simulink model "Engine_TestBench1"  (R2017a)
settings: Solver=ode1  StartTime=0.0  StopTime=1800  FixedStep=0.01  RelTol=1e-3  EnableMultiTasking=on
PostLoadFcn:
  | , if any(exist('dsrtsu_mdlpostloadfcn', 'file') == [2, 3, 6]), try dsrtsu_mdlpostloadfcn('Execute', bdroot); catch fprintf('Error in PostLoadFcn (dsrtsu_mdlpostloadfcn) for model "%s":\n %s\n', bdroot, lasterr); end, end,
undefined symbols (not defined in the file): air, Engine, env, max_vehicle_rad_air_flow, NeutralGear, ParkGear
libraries: simulink x19, EC2_libraries x2
(part 1 of 2)
settings Model: DSRTSU_INTERNAL_RTI_VER=480  DSRTSU_INTERNAL_RTI_TYPE=rti1006  RTICANMMDATA=struct('GeneralSetupData',struct('modelroot','D:\Desktop_files\Clutchless_P2_Model_R2015b','generalsettings',struct('filesettings',struct('destfolder',struct('Name','RTICANMM_FILES','Check',1),'buildfolder',struct('Name','.','Check',1),'AbsDestfolder',struct('Name','D:\Desktop_files\Clutchless_P2_Model_R2015b\RTICANMM_FILES'),'AbsBuildfolder',struct('Name','D:\Desktop_files\Clutchless_P2_Model_R2015b'))),'options',struct('addpaths',1,'rmpaths',1,'addtrcexclusion',logical(1),'cannavigator',struct('checkmonitoring',0),'show_usrtrc',0,'use_usrtrc',0),'advanced',struct('options',[1 1 1 1 1 1 1 1 1 1 1 1 1 1 1 1 1 1 1 1 1 1 1 1 1 1 1 1 1 1 1 1 1 1 1 1 1 1 1 1 1 1 1 1 1 1 1 1 1 1 1 1 1 1 1 1 1 1 1 1 1 1 1 1 1 1 1 1 1 1 1 1 1 1 1 1 1 1 1 1 1 1 1 1 1 1 1 1 1 1 1 1 1 1 1 1 1 1 1 1]),'MPSetup',{{}},'modelname','P2_Parallel_MIL_withTrailer','block','P2_Parallel_MIL_withTrailer'))  DSRTSU_INTERNAL_RTIFPGA=70  SimulationMode=accelerator  Creator=EcoCar  LastModifiedBy=Vraj M
settings DataIOCC: LimitDataPoints=on
settings OptimizationCC: BlockReduction=off  OptimizeBlockIOStorage=off  BufferReuse=off  GlobalBufferReuse=off  ExpressionFolding=off  LocalBlockOutputs=off  EfficientMapNaN2IntZero=off  LifeSpan=inf
settings DebuggingCC: AllowSymbolicDim=off  SFUnexpectedBacktrackingDiag=warning  SFNoUnconditionalDefaultTransitionDiag=warning  SFExecutionAtInitializationDiag=none
settings HardwareCC: ProdBitPerPointer=32  ProdBitPerSizeT=32  ProdBitPerPtrDiffT=32  ProdLargestAtomicInteger=Integer  ProdWordSize=32  ProdHWDeviceType=Custom Processor->Custom  TargetBitPerPointer=64  TargetBitPerSizeT=64  TargetBitPerPtrDiffT=64  TargetLongLongMode=on  TargetIntDivRoundTo=Zero  TargetEndianess=LittleEndian  TargetWordSize=64  TargetHWDeviceType=MATLAB Host  ProdEqTarget=off
settings ModelReferenceCC: PropagateSignalLabelsOutOfModel=off
settings CodeAppCC: MaxIdLength=128
settings GRTTargetCC: TargetLangStandard=C89/C90 (ANSI)  CombineOutputUpdateFcns=off  GRTInterface=on
settings ConfigComp: CovScope=ReferencedModels  CovIncludeTopModel=off  CovMetricSettings=dw  CovHtmlReporting=on  CovSaveCumulativeToWorkspaceVar=on  CovSaveSingleToWorkspaceVar=on  CovExternalEMLEnable=off

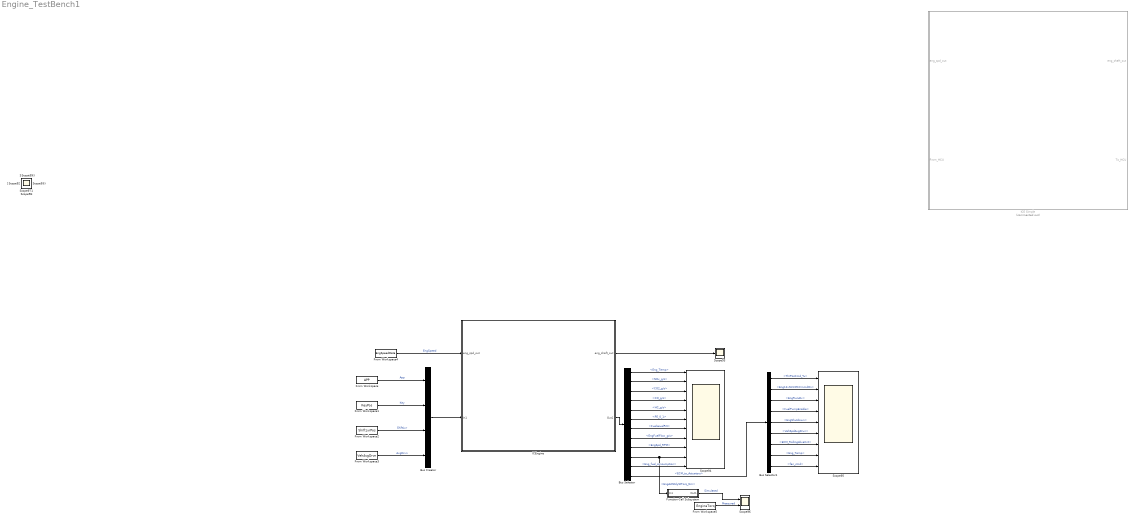
== system Engine_TestBench1 ==
  Bus Creator : BusCreator  Inputs=4
  Bus Selector : BusSelector  OutputSignals=Sensors_to_ECM.Eng_Temp,Sensors_to_ECM.NOx_g/s,Sensors_to_ECM.CO2_g/s,Sensors_to_ECM.CO_g/s,Sensors_to_ECM.HC_g/s,Sensors_to_ECM.PE_0_1,Sensors_to_ECM.FuelLevelPct,Sensors_to_ECM.EngFuelFlow_g/s,Sensors_to_ECM.EngSpd_RPM,Sensors_to_ECM.EngActStdyStTorq_Nm,Eng_fuel_consumption,ECM_to_Actuators
  Bus Selector1 : BusSelector  OutputSignals=ThrPosCmd_%,Eng12vStrtrMtrCmmdOn,EngRunAtv,FuelPumpEnable,EngShutdown,VehSpdAvgDrvn,ECM_RollingAliveCnt,Eng_Temp,fan_cmd
  From Workspace : FromWorkspace  VariableName=APP  SampleTime=0
  From Workspace1 : FromWorkspace  VariableName=KeyPos  SampleTime=0
  From Workspace2 : FromWorkspace  VariableName=ShiftLvrPos  SampleTime=0
  From Workspace3 : FromWorkspace  VariableName=VehAvgDrvn  SampleTime=0
  From Workspace4 : FromWorkspace  VariableName=EngSpeedData  SampleTime=0
  From Workspace5 : FromWorkspace  VariableName=EngineTorq  SampleTime=0
  Function-Call Subsystem : Subsystem  TreatAsAtomicUnit=on
  ICE Simple : Subsystem  Commented=on  AncestorBlock=Engine_simple/ICE Simple
      mask Display:
      | image(imread('EngineTopLevel.jpg'),'center')
      | color('red');
      | port_label('input',1,'SpdOut')
      | port_label('output',1,'ShaftOut')
      | port_label('input',2,'From_HCU')
      | port_label('output',2,'To_HCU')
  ICEngine : Subsystem  AncestorBlock=Engine_simple/ICE Simple
      mask Display:
      | image(imread('EngineTopLevel.jpg'),'center')
      | color('red');
      | port_label('input',1,'SpdOut')
      | port_label('output',1,'ShaftOut')
  Scope{,1..93,97..105} (103 alike) : Scope
  Scope94 : Scope  NumInputPorts=11
  Scope95 : Scope  NumInputPorts=9
  Scope96 : Scope  NumInputPorts=2
  wires:
  Bus Selector1/4 -> Scope95/4  "<FuelPumpEnable>"
  From Workspace2/1 -> Bus Creator/3  "ShiftLvr"
  From Workspace4/1 -> ICEngine/1(eng_spd_out)  "EngSpeed"
  Bus Selector1/7 -> Scope95/7  "<ECM_RollingAliveCnt>"
  ICEngine/2(Out1) -> Bus Selector/1
  Bus Selector1/8 -> Scope95/8  "<Eng_Temp>"
  From Workspace1/1 -> Bus Creator/2  "Key"
  Bus Selector/7 -> Scope94/7  "<FuelLevelPct>"
  Bus Selector/4 -> Scope94/4  "<CO_g/s>"
  Bus Selector/9 -> Scope94/9  "<EngSpd_RPM>"
  Bus Selector/5 -> Scope94/5  "<HC_g/s>"
  Bus Selector/6 -> Scope94/6  "<PE_0_1>"
  Bus Selector/3 -> Scope94/3  "<CO2_g/s>"
  Bus Selector/2 -> Scope94/2  "<NOx_g/s>"
  Bus Selector/10 -> Function-Call Subsystem/1(In1), Scope94/10  "<EngActStdyStTorq_Nm>"
  Bus Selector/11 -> Scope94/11  "<Eng_fuel_consumption>"
  Bus Selector1/6 -> Scope95/6  "<VehSpdAvgDrvn>"
  Bus Creator/1 -> ICEngine/2(In1)
  Bus Selector1/2 -> Scope95/2  "<Eng12vStrtrMtrCmmdOn>"
  Bus Selector1/9 -> Scope95/9  "<fan_cmd>"
  Bus Selector1/1 -> Scope95/1  "<ThrPosCmd_%>"
  Bus Selector1/3 -> Scope95/3  "<EngRunAtv>"
  Bus Selector/1 -> Scope94/1  "<Eng_Temp>"
  From Workspace3/1 -> Bus Creator/4  "AvgDrvn"
  Bus Selector/12 -> Bus Selector1/1  "<ECM_to_Actuators>"
  ICEngine/1(eng_shaft_out) -> Scope93/1
  Bus Selector1/5 -> Scope95/5  "<EngShutdown>"
  Bus Selector/8 -> Scope94/8  "<EngFuelFlow_g/s>"
  From Workspace/1 -> Bus Creator/1  "App"
  From Workspace5/1 -> Scope96/2  "Measured"
  Function-Call Subsystem/1(Out1) -> Scope96/1  "Simulated"

== system Engine_TestBench1/Function-Call Subsystem ==
  In1 : Inport
  Out1 : Outport
  wires:
  In1/1 -> Out1/1  "Simulated"

== system Engine_TestBench1/ICE Simple ==
  eng_spd_out : Inport
  From_HCU : Inport  Port=2
  Engine Plant Modified : Subsystem
      mask Display:
      | image(imread('EngineTopLevel.jpg'),'center')
      | color('red');
      | port_label('input',2,'SpdOut')
      | port_label('output',2,'ShaftOut')
  Soft ECM : Subsystem
      mask Display: image('SoftECU.jpg')
  eng_shaft_out : Outport
  To_HCU : Outport  Port=2
  wires:
  Engine Plant Modified/2(eng_shaft_out) -> eng_shaft_out/1
  eng_spd_out/1 -> Engine Plant Modified/2(eng_spd_out)
  Soft ECM/2(Out1) -> Engine Plant Modified/1("In ")  "ECM_to_Actuators"
  Soft ECM/1(Out) -> To_HCU/1
  Engine Plant Modified/1(Out) -> Soft ECM/2(In1)
  From_HCU/1 -> Soft ECM/1(In)

== system Engine_TestBench1/ICEngine ==
  eng_spd_out : Inport
  In1 : Inport  Port=2
  Engine Plant Modified : Subsystem
      mask Display:
      | image(imread('EngineTopLevel.jpg'),'center')
      | color('red');
      | port_label('input',2,'SpdOut')
      | port_label('output',2,'ShaftOut')
  Soft ECM : Subsystem
      mask Display: image('SoftECU.jpg')
  eng_shaft_out : Outport
  Out1 : Outport  Port=2
  wires:
  Engine Plant Modified/2(eng_shaft_out) -> eng_shaft_out/1
  eng_spd_out/1 -> Engine Plant Modified/2(eng_spd_out)
  Soft ECM/2(Out1) -> Engine Plant Modified/1("In ")  "ECM_to_Actuators"
  In1/1 -> Soft ECM/1(In)
  Soft ECM/1(Out) -> Out1/1
  Engine Plant Modified/1(Out) -> Soft ECM/2(In1)

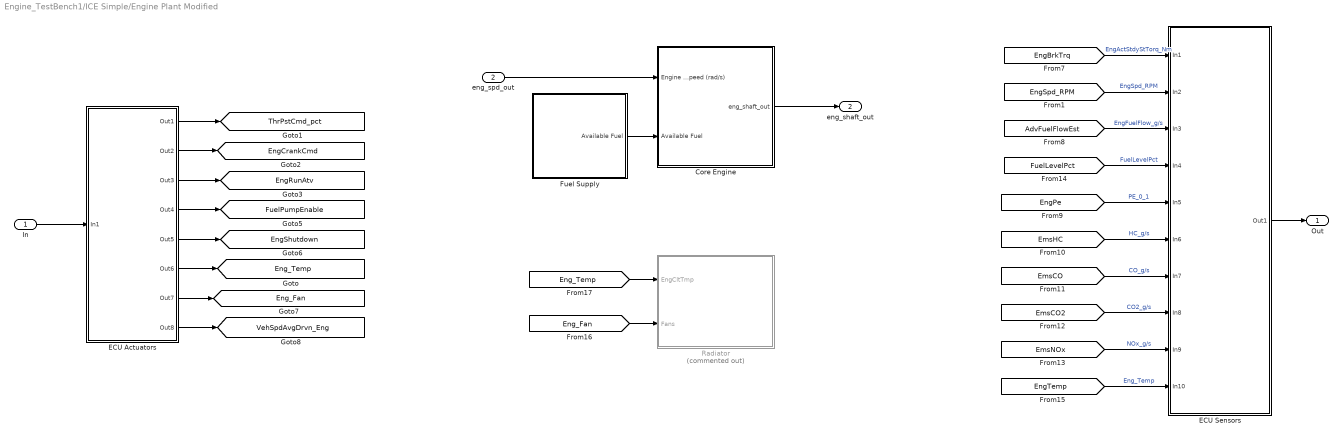
== system Engine_TestBench1/ICE Simple/Engine Plant Modified ==
  "In " : Inport
  eng_spd_out : Inport  Port=2
  Core Engine : Subsystem
      mask Display: image(imread('EngineShortBlock.jpg'),'center')
  ECU Actuators : Subsystem
  ECU Sensors : Subsystem
  Fuel Supply : Subsystem
      mask Display: image(imread('FuelTank.jpg'),'center')
  Radiator : Subsystem  Commented=on  AncestorBlock=lib_Vehicle/Vehicle_Plant_Model/Radiator
  Out : Outport
  eng_shaft_out : Outport  Port=2
  tag scope: EngCrankCmd=global, EngRunAtv=global, EngShutdown=global, Eng_Fan=global, Eng_Temp=global, FuelPumpEnable=global, ThrPstCmd_pct=global, VehSpdAvgDrvn_Eng=global
  wires:
  ECU Actuators/5(Out5) -> [EngShutdown]
  [FuelLevelPct] -> ECU Sensors/4(In4)  "FuelLevelPct"
  [EmsHC] -> ECU Sensors/6(In6)  "HC_g/s"
  [EngPe] -> ECU Sensors/5(In5)  "PE_0_1"
  [EmsCO] -> ECU Sensors/7(In7)  "CO_g/s"
  [EmsCO2] -> ECU Sensors/8(In8)  "CO2_g/s"
  [EmsNOx] -> ECU Sensors/9(In9)  "NOx_g/s"
  Fuel Supply/1(Available Fuel) -> Core Engine/2(Available Fuel)
  ECU Actuators/4(Out4) -> [FuelPumpEnable]
  ECU Actuators/1(Out1) -> [ThrPstCmd_pct]
  "In "/1 -> ECU Actuators/1(In1)
  [EngBrkTrq] -> ECU Sensors/1(In1)  "EngActStdyStTorq_Nm"
  [AdvFuelFlowEst] -> ECU Sensors/3(In3)  "EngFuelFlow_g/s"
  [EngSpd_RPM] -> ECU Sensors/2(In2)  "EngSpd_RPM"
  ECU Actuators/2(Out2) -> [EngCrankCmd]
  ECU Actuators/3(Out3) -> [EngRunAtv]
  Core Engine/1(eng_shaft_out) -> eng_shaft_out/1
  eng_spd_out/1 -> Core Engine/1(Engine Speed (rad/s))
  [EngTemp] -> ECU Sensors/10(In10)  "Eng_Temp"
  [Eng_Fan] -> Radiator/2(Fans)
  [Eng_Temp] -> Radiator/1(EngCltTmp)
  ECU Actuators/6(Out6) -> [Eng_Temp]
  ECU Actuators/7(Out7) -> [Eng_Fan]
  ECU Actuators/8(Out8) -> [VehSpdAvgDrvn_Eng]
  ECU Sensors/1(Out1) -> Out/1

== system Engine_TestBench1/ICE Simple/Soft ECM ==
  note: Should check lookup table with GM
  In : Inport
  In1 : Inport  Port=2
  Bus Creator1 : BusCreator  Inputs=3
  Bus Creator2 : BusCreator  Inputs=9
  Bus Selector : BusSelector  OutputSignals=EngSpd_RPM
  Bus Selector1 : BusSelector  OutputSignals=App,Key,ShiftLvr
  Bus Selector2 : BusSelector  OutputSignals=Eng_Temp,EngFuelFlow_g/s
  Bus Selector3 : BusSelector  OutputSignals=AvgDrvn
  Data Type Conversion : DataTypeConversion  OutDataTypeStr=int8
  Data Type Conversion1 : DataTypeConversion  OutDataTypeStr=int8
  ECM_RollingAliveCnt : Subsystem
  Fuel Consumption : Subsystem
  Logic : Stateflow chart  TreatAsAtomicUnit=on
  Memory1 : Memory  X0=Engine.Init_T_amb
  Memory2 : Memory  InheritSampleTime=on
  Subsystem : Subsystem
  temp vs fan : Lookup_n-D  NumberOfTableDimensions=1  BreakpointsForDimension1=[0:1:100]  Table=[0:0.01:1]  InternalRulePriority=Speed  RndMeth=Simplest  InputSameDT=on
  Out : Outport
  Out1 : Outport  Port=2
  wires:
  Logic/3(EngRunAtv) -> Bus Creator2/3  "EngRunAtv"
  Bus Selector/1 -> Logic/4(EngSpd_RPM)  "<EngSpd_RPM>"
  Bus Selector1/1 -> Memory2/1  "<App>"
  Logic/2(EngCrankCmd) -> Bus Creator2/2  "Eng12vStrtrMtrCmmdOn"
  Bus Creator1/1 -> Out/1  "ECM_CAN"
  Bus Creator2/1 -> Bus Creator1/1, Out1/1  "ECM_to_Actuators"
  Logic/1(ThrottleCmd) -> Bus Creator2/1  "ThrPosCmd_%"
  In1/1 -> Bus Selector/1, Bus Creator1/3, Bus Selector2/1  "Sensors_to_ECM"
  In/1 -> Bus Selector3/1, Bus Selector1/1  "HCU_to_ECM"
  Logic/4(FuelPumpEnable) -> Bus Creator2/4  "FuelPumpEnable"
  Bus Selector1/2 -> Data Type Conversion/1  "<Key>"
  Bus Selector3/1 -> Subsystem/1(In2), Logic/5(VehSpdAvgDrvn)  "<AvgDrvn>"
  Bus Selector1/3 -> Data Type Conversion1/1  "<ShiftLvr>"
  Logic/5(EngShutdown) -> Bus Creator2/5  "EngShutdown"
  Bus Selector2/1 -> temp vs fan/1, Memory1/1  "<Eng_Temp>"
  Bus Selector2/2 -> Fuel Consumption/1(Fuel Consumption)  "<EngFuelFlow_g/s>"
  Fuel Consumption/1(fuel consumption) -> Bus Creator1/2  "Eng_fuel_consumption"
  temp vs fan/1 -> Bus Creator2/9  "fan_cmd"
  Memory1/1 -> Bus Creator2/8  "Eng_Temp"
  Memory2/1 -> Logic/1(drvAPP)
  ECM_RollingAliveCnt/1(Out1) -> Bus Creator2/7
  Data Type Conversion/1 -> Logic/2(SysPwrMd)
  Data Type Conversion1/1 -> Logic/3(ShftLvrPos)
  Subsystem/1(Out1) -> Bus Creator2/6

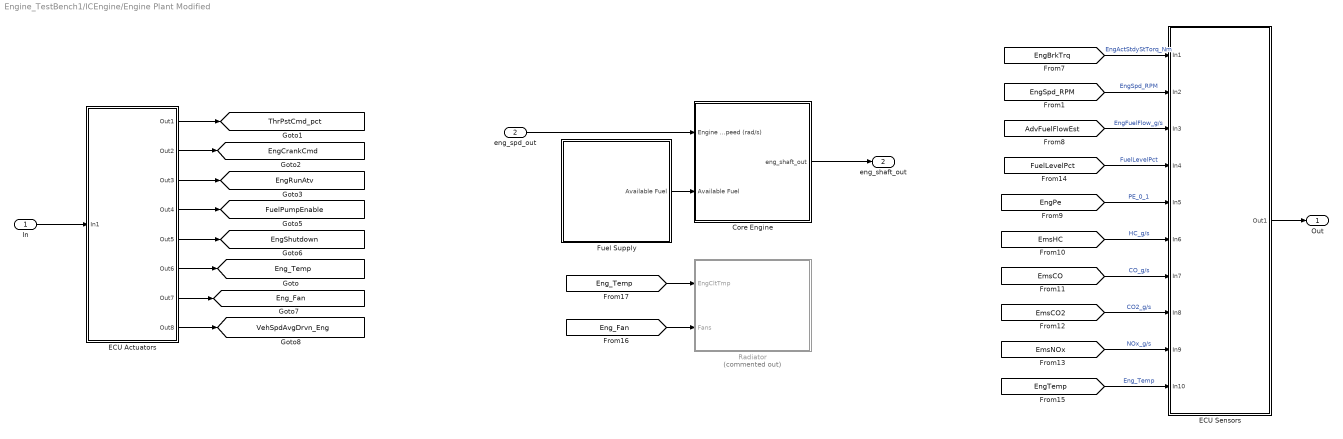
== system Engine_TestBench1/ICEngine/Engine Plant Modified ==
  "In " : Inport
  eng_spd_out : Inport  Port=2
  Core Engine : Subsystem
      mask Display: image(imread('EngineShortBlock.jpg'),'center')
  ECU Actuators : Subsystem
  ECU Sensors : Subsystem
  Fuel Supply : Subsystem
      mask Display: image(imread('FuelTank.jpg'),'center')
  Radiator : Subsystem  Commented=on  AncestorBlock=lib_Vehicle/Vehicle_Plant_Model/Radiator
  Out : Outport
  eng_shaft_out : Outport  Port=2
  tag scope: EngCrankCmd=global, EngRunAtv=global, EngShutdown=global, Eng_Fan=global, Eng_Temp=global, FuelPumpEnable=global, ThrPstCmd_pct=global, VehSpdAvgDrvn_Eng=global
  wires:
  ECU Actuators/5(Out5) -> [EngShutdown]
  [FuelLevelPct] -> ECU Sensors/4(In4)  "FuelLevelPct"
  [EmsHC] -> ECU Sensors/6(In6)  "HC_g/s"
  [EngPe] -> ECU Sensors/5(In5)  "PE_0_1"
  [EmsCO] -> ECU Sensors/7(In7)  "CO_g/s"
  [EmsCO2] -> ECU Sensors/8(In8)  "CO2_g/s"
  [EmsNOx] -> ECU Sensors/9(In9)  "NOx_g/s"
  Fuel Supply/1(Available Fuel) -> Core Engine/2(Available Fuel)
  ECU Actuators/4(Out4) -> [FuelPumpEnable]
  ECU Actuators/1(Out1) -> [ThrPstCmd_pct]
  "In "/1 -> ECU Actuators/1(In1)
  [EngBrkTrq] -> ECU Sensors/1(In1)  "EngActStdyStTorq_Nm"
  [AdvFuelFlowEst] -> ECU Sensors/3(In3)  "EngFuelFlow_g/s"
  [EngSpd_RPM] -> ECU Sensors/2(In2)  "EngSpd_RPM"
  ECU Actuators/2(Out2) -> [EngCrankCmd]
  ECU Actuators/3(Out3) -> [EngRunAtv]
  Core Engine/1(eng_shaft_out) -> eng_shaft_out/1
  eng_spd_out/1 -> Core Engine/1(Engine Speed (rad/s))
  [EngTemp] -> ECU Sensors/10(In10)  "Eng_Temp"
  [Eng_Fan] -> Radiator/2(Fans)
  [Eng_Temp] -> Radiator/1(EngCltTmp)
  ECU Actuators/6(Out6) -> [Eng_Temp]
  ECU Actuators/7(Out7) -> [Eng_Fan]
  ECU Actuators/8(Out8) -> [VehSpdAvgDrvn_Eng]
  ECU Sensors/1(Out1) -> Out/1

== system Engine_TestBench1/ICEngine/Soft ECM ==
  note: Should check lookup table with GM
  In : Inport
  In1 : Inport  Port=2
  Bus Creator1 : BusCreator  Inputs=3
  Bus Creator2 : BusCreator  Inputs=9
  Bus Selector : BusSelector  OutputSignals=EngSpd_RPM
  Bus Selector1 : BusSelector  OutputSignals=App,Key,ShiftLvr
  Bus Selector2 : BusSelector  OutputSignals=Eng_Temp,EngFuelFlow_g/s
  Bus Selector3 : BusSelector  OutputSignals=AvgDrvn
  Data Type Conversion : DataTypeConversion  OutDataTypeStr=int8
  Data Type Conversion1 : DataTypeConversion  OutDataTypeStr=int8
  ECM_RollingAliveCnt : Subsystem
  ECM_RollingAliveCnt1 : Subsystem
  Fuel Consumption : Subsystem
  Logic : Stateflow chart  TreatAsAtomicUnit=on
  Memory1 : Memory  X0=Engine.Init_T_amb
  Memory2 : Memory
  temp vs fan : Lookup_n-D  NumberOfTableDimensions=1  BreakpointsForDimension1=[0:1:100]  Table=[0:0.01:1]  InternalRulePriority=Speed  RndMeth=Simplest  InputSameDT=on
  Out : Outport
  Out1 : Outport  Port=2
  wires:
  Logic/3(EngRunAtv) -> Bus Creator2/3  "EngRunAtv"
  Bus Selector/1 -> Logic/4(EngSpd_RPM)  "<EngSpd_RPM>"
  Bus Selector1/1 -> Memory2/1  "<App>"
  Logic/2(EngCrankCmd) -> Bus Creator2/2  "Eng12vStrtrMtrCmmdOn"
  Bus Creator1/1 -> Out/1  "ECM_CAN"
  Bus Creator2/1 -> Out1/1, Bus Creator1/1  "ECM_to_Actuators"
  Logic/1(ThrottleCmd) -> Bus Creator2/1  "ThrPosCmd_%"
  In1/1 -> Bus Selector2/1, Bus Creator1/3, Bus Selector/1  "Sensors_to_ECM"
  In/1 -> Bus Selector3/1, Bus Selector1/1  "HCU_to_ECM"
  Logic/4(FuelPumpEnable) -> Bus Creator2/4  "FuelPumpEnable"
  Bus Selector1/2 -> Data Type Conversion/1  "<Key>"
  Bus Selector3/1 -> ECM_RollingAliveCnt1/1(In1), Logic/5(VehSpdAvgDrvn)  "<AvgDrvn>"
  Bus Selector1/3 -> Data Type Conversion1/1  "<ShiftLvr>"
  Logic/5(EngShutdown) -> Bus Creator2/5  "EngShutdown"
  Bus Selector2/1 -> Memory1/1, temp vs fan/1  "<Eng_Temp>"
  Bus Selector2/2 -> Fuel Consumption/1(Fuel Consumption)  "<EngFuelFlow_g/s>"
  Fuel Consumption/1(fuel consumption) -> Bus Creator1/2  "Eng_fuel_consumption"
  temp vs fan/1 -> Bus Creator2/9  "fan_cmd"
  Memory1/1 -> Bus Creator2/8  "Eng_Temp"
  ECM_RollingAliveCnt/1(Out1) -> Bus Creator2/7
  Data Type Conversion/1 -> Logic/2(SysPwrMd)
  Data Type Conversion1/1 -> Logic/3(ShftLvrPos)
  Memory2/1 -> Logic/1(drvAPP)
  ECM_RollingAliveCnt1/1(Out1) -> Bus Creator2/6

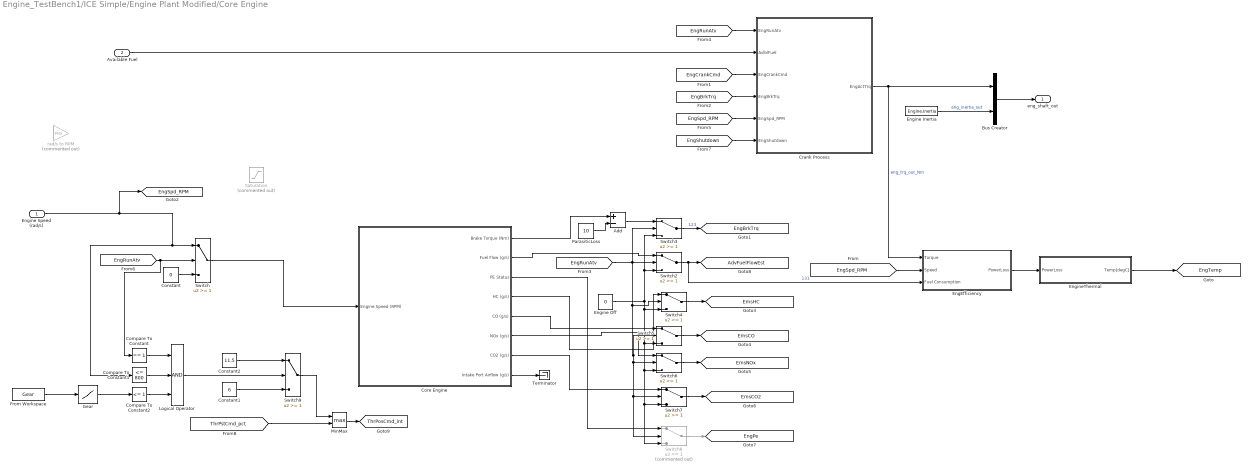
== system Engine_TestBench1/ICE Simple/Engine Plant Modified/Core Engine ==
  Engine Speed (rad/s) : Inport
  Available Fuel : Inport  Port=2
  Add : Sum  Inputs=+-
  Bus Creator : BusCreator  Inputs=2
  Compare To Constant : simulink/Logic and Bit Operations/Compare To Constant  relop===  const=1  OutDataTypeStr=boolean
  Compare To Constant1 : simulink/Logic and Bit Operations/Compare To Constant  relop=<=  const=800  OutDataTypeStr=boolean
  Compare To Constant2 : simulink/Logic and Bit Operations/Compare To Constant  relop=<=  const=1  OutDataTypeStr=boolean
  Constant : Constant  Value=0
  Constant1 : Constant  Value=6
  Constant2 : Constant  Value=11.5
  Core Engine : Subsystem
      mask Display: image(imread('EngineShortBlock.jpg'),'center')
  Crank Process : Stateflow chart  TreatAsAtomicUnit=on
  EngEfficiency : Subsystem
  Engine Inertia : Constant  Value=Engine.Inertia
  "Engine Off  " : Constant  Value=0
  EngineThermal : Subsystem
  From Workspace : FromWorkspace  VariableName=Gear  SampleTime=0
  Gear : Lookup  InputValues=gb.plant.init.gear.idx1_shifter  Table=gb.plant.init.gear.idx2_gear  LookUpMeth=Interpolation-Use End Values  OutDataTypeStr=double  SaturateOnIntegerOverflow=on
  Logical Operator : Logic  Inputs=3  AllPortsSameDT=off  OutDataTypeStr=boolean
  MinMax : MinMax  Function=max  Inputs=2
  ParasiticLoss : Constant  Value=10
  Saturation : Saturate  Commented=on  UpperLimit=max(Engine.Engine.TQ.SPEED)  LowerLimit=0
  Switch{,2..7,9} (8 alike) : Switch  Threshold=1
  Switch8 : Switch  Commented=on  Threshold=1
  Terminator : Terminator
  rad/s to RPM : Gain  Commented=on  Gain=30/pi
  eng_shaft_out : Outport
  tag scope: AdvFuelFlowEst=global, EmsCO2=global, EmsCO=global, EmsHC=global, EmsNOx=global, EngBrkTrq=global, EngPe=global, EngSpd_RPM=global, EngTemp=global, ThrPosCmd_int=global
  wires:
  [EngShutdown] -> Crank Process/6(EngShutdown)
  Engine Speed (rad/s)/1 -> Compare To Constant1/1, Switch/1, [EngSpd_RPM]
  [EngSpd_RPM] -> Crank Process/5(EngSpd_RPM)
  [EngCrankCmd] -> Crank Process/3(EngCrankCmd)
  [EngBrkTrq] -> Crank Process/4(EngBrkTrq)
  [EngRunAtv] -> Crank Process/1(EngRunAtv)
  Switch8/1 -> [EngPe]
  Switch7/1 -> [EmsCO2]
  Switch6/1 -> [EmsNOx]
  Switch5/1 -> [EmsCO]
  "Engine Off  "/1 -> Switch8/3, Switch7/3, Switch6/3, Switch5/3, Switch4/3, Switch2/3, Switch3/3
  [EngRunAtv] -> Switch8/2, Switch7/2, Switch6/2, Switch5/2, Switch4/2, Switch2/2, Switch3/2
  Switch4/1 -> [EmsHC]
  Switch3/1 -> [EngBrkTrq]  "123"
  Available Fuel/1 -> Crank Process/2(AvlblFuel)
  Switch2/1 -> EngEfficiency/3(Fuel Consumption), [AdvFuelFlowEst]  "131"
  Crank Process/1(EngActTrq) -> EngEfficiency/1(Torque), Bus Creator/1  "eng_trq_out_Nm"
  Engine Inertia/1 -> Bus Creator/2  "eng_inertia_out"
  Bus Creator/1 -> eng_shaft_out/1
  [EngRunAtv] -> Switch/2, Compare To Constant/1
  Constant/1 -> Switch/3
  EngEfficiency/1(PowerLoss) -> EngineThermal/1(PowerLoss)
  [EngSpd_RPM] -> EngEfficiency/2(Speed)
  EngineThermal/1(Temp[degC]) -> [EngTemp]
  Core Engine/2(Fuel Flow (g/s)) -> Switch2/1
  Core Engine/3(PE Status) -> Switch8/1
  Core Engine/4(HC (g/s)) -> Switch4/1
  Core Engine/5(CO (g/s)) -> Switch5/1
  Core Engine/6(NOx (g/s)) -> Switch6/1
  Core Engine/7(CO2 (g/s)) -> Switch7/1
  Core Engine/8(Intake Port Airflow (g/s)) -> Terminator/1
  Switch/1 -> Core Engine/1(Engine Speed (RPM))
  Core Engine/1(Brake Torque (Nm)) -> Add/1
  Constant2/1 -> Switch9/1
  Compare To Constant/1 -> Logical Operator/1
  Compare To Constant1/1 -> Logical Operator/2
  Logical Operator/1 -> Switch9/2
  Gear/1 -> Compare To Constant2/1
  Compare To Constant2/1 -> Logical Operator/3
  [ThrPstCmd_pct] -> MinMax/2
  MinMax/1 -> [ThrPosCmd_int]
  Constant1/1 -> Switch9/3
  Switch9/1 -> MinMax/1
  ParasiticLoss/1 -> Add/2
  Add/1 -> Switch3/1
  From Workspace/1 -> Gear/1

== system Engine_TestBench1/ICE Simple/Engine Plant Modified/ECU Actuators ==
  In1 : Inport
  Bus Selector : BusSelector  OutputSignals=ThrPosCmd_%,Eng12vStrtrMtrCmmdOn,EngRunAtv,FuelPumpEnable,EngShutdown,Eng_Temp,fan_cmd,VehSpdAvgDrvn
  Out1 : Outport
  Out2 : Outport  Port=2
  Out3 : Outport  Port=3
  Out4 : Outport  Port=4
  Out5 : Outport  Port=5
  Out6 : Outport  Port=6
  Out7 : Outport  Port=7
  Out8 : Outport  Port=8
  wires:
  Bus Selector/5 -> Out5/1  "<EngShutdown>"
  Bus Selector/4 -> Out4/1  "<FuelPumpEnable>"
  In1/1 -> Bus Selector/1
  Bus Selector/1 -> Out1/1  "<ThrPosCmd_%>"
  Bus Selector/2 -> Out2/1  "<Eng12vStrtrMtrCmmdOn>"
  Bus Selector/3 -> Out3/1  "<EngRunAtv>"
  Bus Selector/6 -> Out6/1  "<Eng_Temp>"
  Bus Selector/7 -> Out7/1  "<fan_cmd>"
  Bus Selector/8 -> Out8/1  "<VehSpdAvgDrvn>"

== system Engine_TestBench1/ICE Simple/Engine Plant Modified/ECU Sensors ==
  In1 : Inport
  In2 : Inport  Port=2
  In3 : Inport  Port=3
  In4 : Inport  Port=4
  In5 : Inport  Port=5
  In6 : Inport  Port=6
  In7 : Inport  Port=7
  In8 : Inport  Port=8
  In9 : Inport  Port=9
  In10 : Inport  Port=10
  Bus Creator : BusCreator  Inputs=10
  Memory : Memory
  Out1 : Outport
  wires:
  In9/1 -> Bus Creator/9  "NOx_g/s"
  In1/1 -> Bus Creator/1  "EngActStdyStTorq_Nm"
  In2/1 -> Bus Creator/2  "EngSpd_RPM"
  In3/1 -> Bus Creator/3  "EngFuelFlow_g/s"
  In4/1 -> Bus Creator/4  "FuelLevelPct"
  In5/1 -> Bus Creator/5  "PE_0_1"
  In6/1 -> Bus Creator/6  "HC_g/s"
  In7/1 -> Bus Creator/7  "CO_g/s"
  Bus Creator/1 -> Memory/1
  In8/1 -> Bus Creator/8  "CO2_g/s"
  In10/1 -> Bus Creator/10  "Eng_Temp"
  Memory/1 -> Out1/1

== system Engine_TestBench1/ICE Simple/Engine Plant Modified/Fuel Supply ==
  0 to 100 : Saturate
  Fuel Pump Disable : Constant  Value=0
  Fuel Volumn : Constant  Value=Engine.Fuel.Initial_Volumn
  Integrator : Integrator  LimitOutput=on  UpperSaturationLimit=Engine.FuelTank.Volume  LowerSaturationLimit=0
  L to % : Gain  Gain=100/Engine.FuelTank.Volume
  Sum : Sum  Inputs=+-
  Switch : Switch  Threshold=1
  g to L : Gain  Gain=1/Engine.Fuel.Density/1000
  Available Fuel : Outport
  tag scope: FuelLevelPct=global
  wires:
  0 to 100/1 -> [FuelLevelPct]
  L to %/1 -> 0 to 100/1
  Fuel Pump Disable/1 -> Switch/3
  g to L/1 -> Switch/1
  Integrator/1 -> g to L/1
  [AdvFuelFlowEst] -> Integrator/1
  [FuelPumpEnable] -> Switch/2
  Sum/1 -> Available Fuel/1, L to %/1
  Switch/1 -> Sum/2
  Fuel Volumn/1 -> Sum/1

== system Engine_TestBench1/ICE Simple/Engine Plant Modified/Radiator ==
  note: Calculation of max air flow:
      |
      | The air flow reach the max in the scenario that only fan rejects all the heat coolant brings in
      |
      | The regular max CFM of a vehicle radiator fan is about 2000
      |
      | CFM=1.76* Q/delta T_air
      |
      | Where Q is the max amount of heat from coolant, assume that the max temperature drop of coolant
      | through radiator is 10 deg C
      |
      | Q= Mc_coolant* Cp_coolant* delta T_coolant=3500*0.26*10=9100w
      |
      | delta T_air=1.76*Q/CFM=1.76*9100/2000=8 degC
      |
      | Max Mc_air=Q/(Cp_air*delta T_air)=9100/(1006*8)=1.13 kg/s
  EngCltTmp : Inport
  Fans : Inport  Port=2
  " " : Product  Inputs=**
  " " : Gain  Gain=0.05
  Ambient Temp : Constant  Value=env.init.T_ambiant
  Compare To Zero : simulink/Logic and Bit Operations/Compare To Zero  relop=<=  OutDataTypeStr=boolean
  Constant : Constant
  Cp of Air : Constant  Value=air.init.specific_heat
  Cp of Air1 : Constant  Value=air.init.specific_heat
  Data Type Conversion1 : DataTypeConversion
  Divide by Zero Fix : Subsystem
  "Eng Mc=Q/(Cp*delta T) " : Product  Inputs=*/
  Q=Mc_air*Cp_air*delta T : Product  Inputs=***
  Saturation : Saturate  UpperLimit=max_vehicle_rad_air_flow  LowerLimit=-1
  Sum3 : Sum  Inputs=|-+
  Sum4 : Sum
  Sum5 : Sum  Inputs=|+-
  Switch : Switch  Threshold=1
  vehspdflow : Gain  Gain=0.01
  tag scope: AirFlowRequest=global, Heat_Reject_Eng=global
  wires:
  Data Type Conversion1/1 -> " "/1
  Cp of Air1/1 -> Q=Mc_air*Cp_air*delta T/3
  Switch/1 -> Q=Mc_air*Cp_air*delta T/2  "eng act air flow in kg/s"
  Q=Mc_air*Cp_air*delta T/1 -> " "/2  "J/s"
  " "/1 -> [Heat_Reject_Eng]  "J"
  Saturation/1 -> Sum3/1  "Actual air flow"
  Sum3/1 -> Compare To Zero/1
  Compare To Zero/1 -> Switch/2  "request meet"
  Cp of Air/1 -> "Eng Mc=Q/(Cp*delta T) "/2  "Cp J/kg*C"
  Ambient Temp/1 -> Sum5/2  "25 deg C"
  Sum5/1 -> Divide by Zero Fix/2(Divide), Q=Mc_air*Cp_air*delta T/1  "Delta T = Tcoolant - Tambient"
  EngCltTmp/1 -> Sum5/1  "EngCltTmp in deg C"
  "Eng Mc=Q/(Cp*delta T) "/1 -> Switch/1, Sum3/2, [AirFlowRequest]  "Eng requested air flow in Kg/s"
  Sum4/1 -> Switch/3, Saturation/1  "Air Flow Recieved"
  Fans/1 -> Data Type Conversion1/1
  [VehSpdAvgDrvn_Eng] -> vehspdflow/1
  vehspdflow/1 -> Sum4/2
  [Heat_Transfer_Eng_1] -> Divide by Zero Fix/1(Multiply)  "heat generation in w"
  Divide by Zero Fix/1(Output) -> "Eng Mc=Q/(Cp*delta T) "/1
  " "/1 -> Sum4/1
  Constant/1 -> " "/1

== system Engine_TestBench1/ICE Simple/Soft ECM/ECM_RollingAliveCnt ==
  Constant : Constant
  Rolling Alive Counter : Stateflow chart  TreatAsAtomicUnit=on
  Switch : Switch  Criteria=u2 > Threshold
  Out1 : Outport
  wires:
  [ECM_CAN_fault] -> Switch/2
  Constant/1 -> Switch/1
  Rolling Alive Counter/1(RollingAliveCnt) -> Switch/3
  Switch/1 -> Out1/1  "ECM_RollingAliveCnt"

== system Engine_TestBench1/ICE Simple/Soft ECM/Fuel Consumption ==
  note: Total Fuel Consumed
  Fuel Consumption : Inport
  " " : Constant  Value=3600
  " tloop" : Constant  Value=0.01
  1/fuel density : Gain  Gain=1/(Engine.Fuel.Density*1000)
  Add : Sum  Inputs=|++
  Add1 : Sum  Inputs=|++
  Constant3 : Constant  Value=Engine.Fuel.Lower_Heating_Value/1000
  Divide : Product  Inputs=*/
  Divide by Zero Fix : Subsystem
  Divide by Zero Fix1 : Subsystem
  Memory : Memory
  Memory1 : Memory
  Product : Product  RndMeth=Zero
  Product1 : Product  RndMeth=Zero
  Product3 : Product  RndMeth=Zero
  Scope : Scope
  To Workspace5 : ToWorkspace  Commented=on  VariableName=eng_wh_per_mile_hist  SampleTime=-1
      settings: Decimation=WORKSPACE_DECIMATION
  fuel consumption : Outport
  wires:
  Divide by Zero Fix1/1(Output) -> To Workspace5/1
  Divide/1 -> Add1/1  "Wh"
  Memory1/1 -> Add1/2
  Add1/1 -> Divide by Zero Fix1/2(Multiply), Memory1/1  "cumulative"
  Product/1 -> Product3/2  "W"
  Constant3/1 -> Product/2
  Divide by Zero Fix/1(Output) -> fuel consumption/1, Scope/1
  [veh_dist_miles] -> Divide by Zero Fix1/1(Divide), Divide by Zero Fix/2(Multiply)  "miles"
  Product1/1 -> Add/1  "liter"
  1/fuel density/1 -> Product1/1  "liter/sec"
  Fuel Consumption/1 -> Product/1, 1/fuel density/1  "g/s"
  Memory/1 -> Add/2
  Add/1 -> Divide by Zero Fix/1(Divide), Memory/1  "cumulative_liter"
  " tloop"/1 -> Product3/1, Product1/2
  Product3/1 -> Divide/1
  " "/1 -> Divide/2

== system Engine_TestBench1/ICE Simple/Soft ECM/Logic/APP2TP ==
  EngSpd : Inport
  APP : Inport  Port=2
  Shifter : Inport  Port=3
  f : TriggerPort  TriggerType=function-call  VariantControl=Variant
      settings: CopyFcn=Stateflow.SLINSF.SimulinkMan.removeBlockPreDeleteFcn  PreDeleteFcn=Stateflow.SLINSF.SimulinkMan.unsafePredeleteFcn
  Based on APP to TP test data from 2013 Malibu : Lookup_n-D  NumberOfTableDimensions=1  BreakpointsForDimension1=[0,1,2,3,4,5,6,7,8,9,10,11,12,13,14,15,16,17,18,19,20,21,22,23,24,25,26,27,28,29,30,31,32,33,34,35,36,37,38,39,40,41,42,43,44,45,46,48,51,55,60,66,100]  Table=[0,6.3,12.7686537241448,12.6326703204763,12.8888951657611,13.4307541011932,14.1739282202018,15.0532596030224,16.0198646102832,17.0384547356068,18.0848650172271,19.1437900086214,20.206727308158,21.2701286477589,22.3337585405773,23.3992604876916,24.4689307438132,25.5446996420107,26.6273204774486,27.7157659501418,28.8068321667249,29.8949502012373,30.9722052149229,32.0285631350456,33.0523048927199,34.0306682197568,34.9506970045247,35.8002982068255,36.5695063317874,37.2519554627699,37.846558853288,38.359396077948,38.8058077424007,39.2126977523099,39.6210431413345,40.0886114581279,40.6928857123509,41.5341968797017,42.7390639659588,44.4637416300428,46.8979753660875,50.2689642445339,54.8455312122302,60.9425009515619,68.9252852985734,79.2146762201353,81.9427,84.6943,87.2166,89.5096,91.3439,92.6051,100]  ExtrapMethod=Clip  UseLastTableValue=on  InternalRulePriority=Speed  RndMeth=Simplest  InputSameDT=on
  Compare To Constant : simulink/Logic and Bit Operations/Compare To Constant  relop=<=  const=Engine.IdleSpeed  OutDataTypeStr=boolean
  Compare To Constant1 : simulink/Logic and Bit Operations/Compare To Constant  relop=<=  const=3.0  OutDataTypeStr=boolean
  Constant : Constant  Value=ParkGear
  Constant1 : Constant  Value=NeutralGear
  Constant2 : Constant  Value=Engine.IdleSpeed
  Display : Display
  Divide : Product  Inputs=**
  "EngSpd " : InportShadow
  Kp : Gain  Gain=0.5
  Logical Operator : Logic  Operator=OR  Inputs=3  AllPortsSameDT=off  OutDataTypeStr=boolean
  Logical Operator1 : Logic  AllPortsSameDT=off  OutDataTypeStr=boolean
  Memory : Memory  InheritSampleTime=on
  Product : Product
  RPM Derating : Lookup_n-D  NumberOfTableDimensions=1  BreakpointsForDimension1=[0 1000 2000 3000 4000 5000 6000 7000]  Table=[1 1 1 1 1 1 1 0]  ExtrapMethod=Clip  UseLastTableValue=on  InternalRulePriority=Speed  RndMeth=Simplest  InputSameDT=on
  Relational Operator : RelationalOperator  Operator===  OutDataTypeStr=boolean  RndMeth=Nearest
  Relational Operator1 : RelationalOperator  Operator===  OutDataTypeStr=boolean  RndMeth=Nearest
  Sum : Sum  Inputs=|+-
  Switch : Switch  Threshold=1
  TP : Outport
  wires:
  Based on APP to TP test data from 2013 Malibu/1 -> Product/1  "1"
  EngSpd/1 -> Compare To Constant/1, RPM Derating/1
  RPM Derating/1 -> Product/2  "2"
  Shifter/1 -> Relational Operator/2, Relational Operator1/1
  Constant/1 -> Relational Operator/1
  Constant1/1 -> Relational Operator1/2
  Relational Operator/1 -> Logical Operator/1
  Relational Operator1/1 -> Logical Operator/2
  Logical Operator/1 -> Logical Operator1/1
  Constant2/1 -> Sum/1
  "EngSpd "/1 -> Sum/2
  Sum/1 -> Divide/2
  Divide/1 -> Memory/1, Switch/1
  Logical Operator1/1 -> ?  "Idle"
  Compare To Constant1/1 -> Logical Operator1/2
  APP/1 -> Display/1, Compare To Constant1/1, Based on APP to TP test data from 2013 Malibu/1  "3"
  Product/1 -> Switch/3
  Compare To Constant/1 -> Logical Operator/3
  Switch/1 -> TP/1
  Memory/1 -> Kp/1
  Kp/1 -> Divide/1

== system Engine_TestBench1/ICE Simple/Soft ECM/Subsystem ==
  In2 : Inport
  Out1 : Outport
  wires:
  In2/1 -> Out1/1  "VehSpdAvgDrvn"

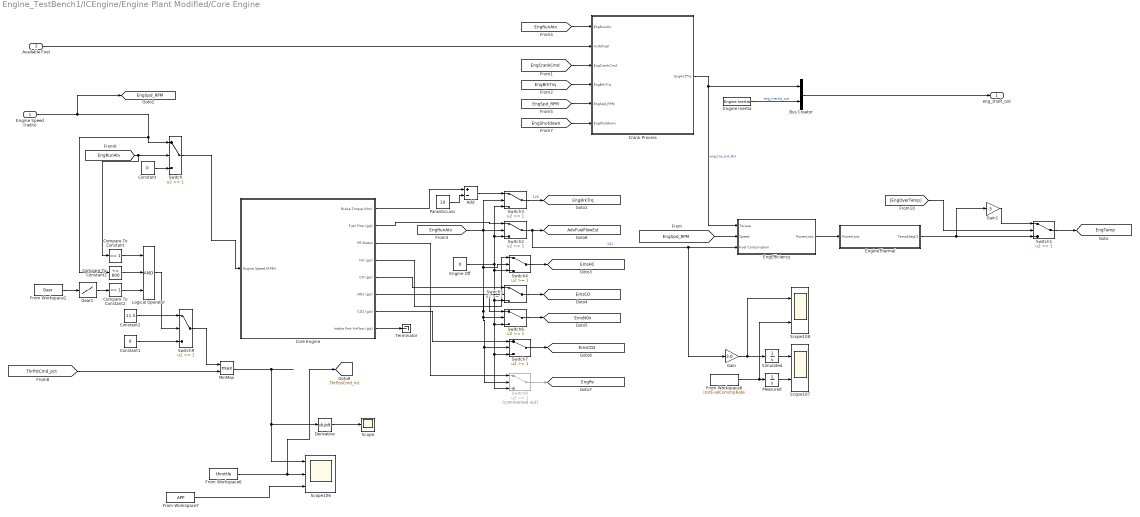
== system Engine_TestBench1/ICEngine/Engine Plant Modified/Core Engine ==
  Engine Speed (rad/s) : Inport
  Available Fuel : Inport  Port=2
  Add : Sum  Inputs=+-
  Bus Creator : BusCreator  Inputs=2
  Compare To Constant : simulink/Logic and Bit Operations/Compare To Constant  relop===  const=1  OutDataTypeStr=boolean
  Compare To Constant1 : simulink/Logic and Bit Operations/Compare To Constant  relop=<=  const=800  OutDataTypeStr=boolean
  Compare To Constant2 : simulink/Logic and Bit Operations/Compare To Constant  relop=<=  const=1  OutDataTypeStr=boolean
  Constant : Constant  Value=0
  Constant1 : Constant  Value=6
  Constant2 : Constant  Value=11.5
  Core Engine : Subsystem
      mask Display: image(imread('EngineShortBlock.jpg'),'center')
  Crank Process : Stateflow chart  TreatAsAtomicUnit=on
  Derivative : Derivative
  EngEfficiency : Subsystem
  Engine Inertia : Constant  Value=Engine.Inertia
  "Engine Off  " : Constant  Value=0
  EngineThermal : Subsystem
  From Workspace2 : FromWorkspace  VariableName=Gear  SampleTime=0
  From Workspace6 : FromWorkspace  VariableName=throttle  SampleTime=0
  From Workspace7 : FromWorkspace  VariableName=APP  SampleTime=0
  From Workspace8 : FromWorkspace  VariableName=InstFuelConsmpRate  SampleTime=0
  Gain : Gain  Gain=3.6
  Gain1 : Gain  Gain=3
  Gear1 : Lookup  InputValues=gb.plant.init.gear.idx1_shifter  Table=gb.plant.init.gear.idx2_gear  LookUpMeth=Interpolation-Use End Values  OutDataTypeStr=double  SaturateOnIntegerOverflow=on
  Logical Operator : Logic  Inputs=3  AllPortsSameDT=off  OutDataTypeStr=boolean
  Measured : Integrator
  MinMax : MinMax  Function=max  Inputs=2
  ParasiticLoss : Constant  Value=10
  Scope : Scope
  Scope106 : Scope  NumInputPorts=3
  Scope107 : Scope  NumInputPorts=2
  Scope108 : Scope  NumInputPorts=2
  Simulated : Integrator
  Switch{,1..7,9} (9 alike) : Switch  Threshold=1
  Switch8 : Switch  Commented=on  Threshold=1
  Terminator : Terminator
  eng_shaft_out : Outport
  tag scope: AdvFuelFlowEst=global, EmsCO2=global, EmsCO=global, EmsHC=global, EmsNOx=global, EngBrkTrq=global, EngPe=global, EngSpd_RPM=global, EngTemp=global, ThrPosCmd_int=global
  wires:
  [EngShutdown] -> Crank Process/6(EngShutdown)
  Engine Speed (rad/s)/1 -> Compare To Constant1/1, Switch/1, [EngSpd_RPM]
  [EngSpd_RPM] -> Crank Process/5(EngSpd_RPM)
  [EngCrankCmd] -> Crank Process/3(EngCrankCmd)
  [EngBrkTrq] -> Crank Process/4(EngBrkTrq)
  [EngRunAtv] -> Crank Process/1(EngRunAtv)
  Switch8/1 -> [EngPe]
  Switch7/1 -> [EmsCO2]
  Switch6/1 -> [EmsNOx]
  Switch5/1 -> [EmsCO]
  "Engine Off  "/1 -> Switch8/3, Switch7/3, Switch6/3, Switch5/3, Switch4/3, Switch2/3, Switch3/3
  [EngRunAtv] -> Switch8/2, Switch7/2, Switch6/2, Switch5/2, Switch4/2, Switch2/2, Switch3/2
  Switch4/1 -> [EmsHC]
  Switch3/1 -> [EngBrkTrq]  "123"
  Available Fuel/1 -> Crank Process/2(AvlblFuel)
  Crank Process/1(EngActTrq) -> Bus Creator/1, EngEfficiency/1(Torque)  "eng_trq_out_Nm"
  Engine Inertia/1 -> Bus Creator/2  "eng_inertia_out"
  Bus Creator/1 -> eng_shaft_out/1
  [EngRunAtv] -> Switch/2, Compare To Constant/1
  Constant/1 -> Switch/3
  EngEfficiency/1(PowerLoss) -> EngineThermal/1(PowerLoss)
  EngineThermal/1(Temp[degC]) -> Gain1/1, Switch1/3
  [EngSpd_RPM] -> EngEfficiency/2(Speed)
  [EngOverTemp] -> Switch1/2
  Gain1/1 -> Switch1/1
  Switch1/1 -> [EngTemp]
  Core Engine/2(Fuel Flow (g/s)) -> Switch2/1
  Core Engine/3(PE Status) -> Switch8/1
  Core Engine/4(HC (g/s)) -> Switch4/1
  Core Engine/5(CO (g/s)) -> Switch5/1
  Core Engine/6(NOx (g/s)) -> Switch6/1
  Core Engine/7(CO2 (g/s)) -> Switch7/1
  Core Engine/8(Intake Port Airflow (g/s)) -> Terminator/1
  Switch/1 -> Core Engine/1(Engine Speed (RPM))
  Core Engine/1(Brake Torque (Nm)) -> Add/1
  Constant2/1 -> Switch9/1
  Compare To Constant/1 -> Logical Operator/1
  Compare To Constant1/1 -> Logical Operator/2
  Logical Operator/1 -> Switch9/2
  Gear1/1 -> Compare To Constant2/1
  Compare To Constant2/1 -> Logical Operator/3
  [ThrPstCmd_pct] -> MinMax/2
  Constant1/1 -> Switch9/3
  Switch9/1 -> MinMax/1
  ParasiticLoss/1 -> Add/2
  Add/1 -> Switch3/1
  From Workspace2/1 -> Gear1/1
  From Workspace6/1 -> [ThrPosCmd_int], Scope106/2
  From Workspace7/1 -> Scope106/3
  Simulated/1 -> Scope107/1
  Measured/1 -> Scope107/2
  Switch2/1 -> Gain/1, EngEfficiency/3(Fuel Consumption), [AdvFuelFlowEst]  "131"
  From Workspace8/1 -> Scope108/2, Measured/1
  Gain/1 -> Scope108/1, Simulated/1
  MinMax/1 -> Derivative/1, Scope106/1
  Derivative/1 -> Scope/1

== system Engine_TestBench1/ICEngine/Engine Plant Modified/ECU Actuators ==
  In1 : Inport
  Bus Selector : BusSelector  OutputSignals=ThrPosCmd_%,Eng12vStrtrMtrCmmdOn,EngRunAtv,FuelPumpEnable,EngShutdown,Eng_Temp,fan_cmd,VehSpdAvgDrvn
  Out1 : Outport
  Out2 : Outport  Port=2
  Out3 : Outport  Port=3
  Out4 : Outport  Port=4
  Out5 : Outport  Port=5
  Out6 : Outport  Port=6
  Out7 : Outport  Port=7
  Out8 : Outport  Port=8
  wires:
  Bus Selector/5 -> Out5/1  "<EngShutdown>"
  Bus Selector/4 -> Out4/1  "<FuelPumpEnable>"
  In1/1 -> Bus Selector/1
  Bus Selector/1 -> Out1/1  "<ThrPosCmd_%>"
  Bus Selector/2 -> Out2/1  "<Eng12vStrtrMtrCmmdOn>"
  Bus Selector/3 -> Out3/1  "<EngRunAtv>"
  Bus Selector/6 -> Out6/1  "<Eng_Temp>"
  Bus Selector/7 -> Out7/1  "<fan_cmd>"
  Bus Selector/8 -> Out8/1  "<VehSpdAvgDrvn>"

== system Engine_TestBench1/ICEngine/Engine Plant Modified/ECU Sensors ==
  In1 : Inport
  In2 : Inport  Port=2
  In3 : Inport  Port=3
  In4 : Inport  Port=4
  In5 : Inport  Port=5
  In6 : Inport  Port=6
  In7 : Inport  Port=7
  In8 : Inport  Port=8
  In9 : Inport  Port=9
  In10 : Inport  Port=10
  Bus Creator : BusCreator  Inputs=10
  Memory : Memory
  Out1 : Outport
  wires:
  In9/1 -> Bus Creator/9  "NOx_g/s"
  In1/1 -> Bus Creator/1  "EngActStdyStTorq_Nm"
  In2/1 -> Bus Creator/2  "EngSpd_RPM"
  In3/1 -> Bus Creator/3  "EngFuelFlow_g/s"
  In4/1 -> Bus Creator/4  "FuelLevelPct"
  In5/1 -> Bus Creator/5  "PE_0_1"
  In6/1 -> Bus Creator/6  "HC_g/s"
  In7/1 -> Bus Creator/7  "CO_g/s"
  Bus Creator/1 -> Memory/1
  In8/1 -> Bus Creator/8  "CO2_g/s"
  In10/1 -> Bus Creator/10  "Eng_Temp"
  Memory/1 -> Out1/1

== system Engine_TestBench1/ICEngine/Engine Plant Modified/Fuel Supply ==
  0 to 100 : Saturate
  Fuel Pump Disable : Constant  Value=0
  Fuel Volumn : Constant  Value=Engine.Fuel.Initial_Volumn
  Integrator : Integrator  LimitOutput=on  UpperSaturationLimit=Engine.FuelTank.Volume  LowerSaturationLimit=0
  L to % : Gain  Gain=100/Engine.FuelTank.Volume
  Sum : Sum  Inputs=+-
  Switch : Switch  Threshold=1
  g to L : Gain  Gain=1/Engine.Fuel.Density/1000
  Available Fuel : Outport
  tag scope: FuelLevelPct=global
  wires:
  0 to 100/1 -> [FuelLevelPct]
  L to %/1 -> 0 to 100/1
  Fuel Pump Disable/1 -> Switch/3
  g to L/1 -> Switch/1
  Integrator/1 -> g to L/1
  [AdvFuelFlowEst] -> Integrator/1
  [FuelPumpEnable] -> Switch/2
  Sum/1 -> Available Fuel/1, L to %/1
  Switch/1 -> Sum/2
  Fuel Volumn/1 -> Sum/1

== system Engine_TestBench1/ICEngine/Engine Plant Modified/Radiator ==
  note: Calculation of max air flow:
      |
      | The air flow reach the max in the scenario that only fan rejects all the heat coolant brings in
      |
      | The regular max CFM of a vehicle radiator fan is about 2000
      |
      | CFM=1.76* Q/delta T_air
      |
      | Where Q is the max amount of heat from coolant, assume that the max temperature drop of coolant
      | through radiator is 10 deg C
      |
      | Q= Mc_coolant* Cp_coolant* delta T_coolant=3500*0.26*10=9100w
      |
      | delta T_air=1.76*Q/CFM=1.76*9100/2000=8 degC
      |
      | Max Mc_air=Q/(Cp_air*delta T_air)=9100/(1006*8)=1.13 kg/s
  EngCltTmp : Inport
  Fans : Inport  Port=2
  " " : Product  Inputs=**
  " " : Gain  Gain=0.05
  Ambient Temp : Constant  Value=env.init.T_ambiant
  Compare To Zero : simulink/Logic and Bit Operations/Compare To Zero  relop===  OutDataTypeStr=uint8
  Constant : Constant
  Cp of Air : Constant  Value=air.init.specific_heat
  Cp of Air1 : Constant  Value=air.init.specific_heat
  Data Type Conversion1 : DataTypeConversion
  Divide by Zero Fix : Subsystem
  "Eng Mc=Q/(Cp*delta T) " : Product  Inputs=*/
  Q=Mc_air*Cp_air*delta T : Product  Inputs=***
  Saturation : Saturate  UpperLimit=max_vehicle_rad_air_flow  LowerLimit=-1
  Sum3 : Sum  Inputs=|-+
  Sum4 : Sum
  Sum5 : Sum  Inputs=|+-
  Switch : Switch  Threshold=1
  vehspdflow : Gain  Gain=0.01
  tag scope: AirFlowRequest=global, Heat_Reject_Eng=global
  wires:
  Data Type Conversion1/1 -> " "/1
  Cp of Air1/1 -> Q=Mc_air*Cp_air*delta T/3
  Switch/1 -> Q=Mc_air*Cp_air*delta T/2  "eng act air flow in kg/s"
  Q=Mc_air*Cp_air*delta T/1 -> " "/2  "J/s"
  " "/1 -> [Heat_Reject_Eng]  "J"
  Saturation/1 -> Sum3/1  "Actual air flow"
  Sum3/1 -> Compare To Zero/1
  Compare To Zero/1 -> Switch/2  "request meet"
  Cp of Air/1 -> "Eng Mc=Q/(Cp*delta T) "/2  "Cp J/kg*C"
  Ambient Temp/1 -> Sum5/2  "25 deg C"
  Sum5/1 -> Divide by Zero Fix/2(Divide), Q=Mc_air*Cp_air*delta T/1  "Delta T = Tcoolant - Tambient"
  EngCltTmp/1 -> Sum5/1  "EngCltTmp in deg C"
  "Eng Mc=Q/(Cp*delta T) "/1 -> Switch/1, Sum3/2, [AirFlowRequest]  "Eng requested air flow in Kg/s"
  Sum4/1 -> Switch/3, Saturation/1  "Air Flow Recieved"
  Fans/1 -> Data Type Conversion1/1
  [VehSpdAvgDrvn_Eng] -> vehspdflow/1
  vehspdflow/1 -> Sum4/2
  [Heat_Transfer_Eng] -> Divide by Zero Fix/1(Multiply)  "heat generation in w"
  Divide by Zero Fix/1(Output) -> "Eng Mc=Q/(Cp*delta T) "/1
  " "/1 -> Sum4/1
  Constant/1 -> " "/1

== system Engine_TestBench1/ICEngine/Soft ECM/ECM_RollingAliveCnt ==
  Constant : Constant
  Rolling Alive Counter : Stateflow chart  TreatAsAtomicUnit=on
  Switch : Switch  Criteria=u2 > Threshold
  Out1 : Outport
  wires:
  [ECM_CAN_fault] -> Switch/2
  Constant/1 -> Switch/1
  Rolling Alive Counter/1(RollingAliveCnt) -> Switch/3
  Switch/1 -> Out1/1  "ECM_RollingAliveCnt"

== system Engine_TestBench1/ICEngine/Soft ECM/ECM_RollingAliveCnt1 ==
  In1 : Inport
  Out1 : Outport
  wires:
  In1/1 -> Out1/1  "VehSpdAvgDrvn"

== system Engine_TestBench1/ICEngine/Soft ECM/Fuel Consumption ==
  note: Total Fuel Consumed
  Fuel Consumption : Inport
  " " : Constant  Value=3600
  " tloop" : Constant  Value=0.001
  1/fuel density : Gain  Gain=1/(Engine.Fuel.Density)
  Add : Sum  Inputs=|++
  Add1 : Sum  Inputs=|++
  Constant3 : Constant  Value=Engine.Fuel.Lower_Heating_Value/1000
  Display2 : Display
  Display3 : Display
  Divide : Product  Inputs=*/
  Divide by Zero Fix : Subsystem
  Divide by Zero Fix1 : Subsystem
  Gain1 : Gain  Gain=0.264172
  Memory : Memory
  Memory1 : Memory
  Product : Product  RndMeth=Zero
  Product1 : Product  RndMeth=Zero
  Product3 : Product  RndMeth=Zero
  Scope : Scope
  To Workspace3 : ToWorkspace  VariableName=eng_fuel_l1  SampleTime=-1
      settings: Decimation=WORKSPACE_DECIMATION
  To Workspace4 : ToWorkspace  VariableName=eng_fuel_gal1  SampleTime=-1
      settings: Decimation=WORKSPACE_DECIMATION
  To Workspace5 : ToWorkspace  VariableName=eng_wh_per_mile_hist  SampleTime=-1
      settings: Decimation=WORKSPACE_DECIMATION
  g/s to Kg/s : Gain  Gain=0.001
  fuel consumption : Outport
  wires:
  Divide by Zero Fix1/1(Output) -> To Workspace5/1
  Divide/1 -> Add1/1  "Wh"
  Memory1/1 -> Add1/2
  Add1/1 -> Divide by Zero Fix1/2(Multiply), Memory1/1  "cumulative"
  Product/1 -> Product3/2  "W"
  Constant3/1 -> Product/2
  Divide by Zero Fix/1(Output) -> fuel consumption/1, Scope/1
  [veh_dist_miles] -> Divide by Zero Fix1/1(Divide), Divide by Zero Fix/2(Multiply)  "miles"
  Product1/1 -> Add/1  "liter"
  1/fuel density/1 -> Product1/1  "liter/sec"
  Fuel Consumption/1 -> g/s to Kg/s/1, Product/1  "g/s"
  Memory/1 -> Add/2
  Add/1 -> Divide by Zero Fix/1(Divide), To Workspace3/1, Gain1/1, Display3/1, Memory/1  "cumulative_liter"
  " tloop"/1 -> Product3/1, Product1/2
  Product3/1 -> Divide/1
  " "/1 -> Divide/2
  g/s to Kg/s/1 -> 1/fuel density/1
  Gain1/1 -> Display2/1, To Workspace4/1

== system Engine_TestBench1/ICEngine/Soft ECM/Logic/APP2TP ==
  EngSpd : Inport
  APP : Inport  Port=2
  Shifter : Inport  Port=3
  f : TriggerPort  TriggerType=function-call  VariantControl=Variant
      settings: CopyFcn=Stateflow.SLINSF.SimulinkMan.removeBlockPreDeleteFcn  PreDeleteFcn=Stateflow.SLINSF.SimulinkMan.unsafePredeleteFcn
  Based on APP to TP test data from 2013 Malibu : Lookup_n-D  NumberOfTableDimensions=1  BreakpointsForDimension1=[0,1,2,3,4,5,6,7,8,9,10,11,12,13,14,15,16,17,18,19,20,21,22,23,24,25,26,27,28,29,30,31,32,33,34,35,36,37,38,39,40,41,42,43,44,45,46,48,51,55,60,66,100]  Table=[0,6.3,12.7686537241448,12.6326703204763,12.8888951657611,13.4307541011932,14.1739282202018,15.0532596030224,16.0198646102832,17.0384547356068,18.0848650172271,19.1437900086214,20.206727308158,21.2701286477589,22.3337585405773,23.3992604876916,24.4689307438132,25.5446996420107,26.6273204774486,27.7157659501418,28.8068321667249,29.8949502012373,30.9722052149229,32.0285631350456,33.0523048927199,34.0306682197568,34.9506970045247,35.8002982068255,36.5695063317874,37.2519554627699,37.846558853288,38.359396077948,38.8058077424007,39.2126977523099,39.6210431413345,40.0886114581279,40.6928857123509,41.5341968797017,42.7390639659588,44.4637416300428,46.8979753660875,50.2689642445339,54.8455312122302,60.9425009515619,68.9252852985734,79.2146762201353,81.9427,84.6943,87.2166,89.5096,91.3439,92.6051,100]  ExtrapMethod=Clip  UseLastTableValue=on  InternalRulePriority=Speed  RndMeth=Simplest  InputSameDT=on
  Based on APP to TP test data from 2013 Malibu1 : Lookup_n-D  NumberOfTableDimensions=1  BreakpointsForDimension1=[0,1,2,3,4,5,6,7,8,9,10,11,12,13,14,15,16,17,18,19,20,21,22,23,24,25,26,27,28,29,30,31,32,33,34,35,36,37,38,39,40,41,42,43,44,45,46,48,51,55,60,66,100]  Table=[7,12,14,16,18,20,22,24,26,28,30,30.33,30.66,31,33,35,36,37,38,39,40,41,42,46,49,51,53,55,57,59,60,62,65,69,72,73,76,79,81,83,85,85.5,86,87,88,89,89.5,90,90.5,91,91.5,93,100]  ExtrapMethod=Clip  UseLastTableValue=on  InputSameDT=on
  Compare To Constant1 : simulink/Logic and Bit Operations/Compare To Constant  relop=<  const=1  OutDataTypeStr=boolean
  Constant : Constant  Value=ParkGear
  Constant1 : Constant  Value=NeutralGear
  Constant2 : Constant  Value=Engine.IdleSpeed
  Display : Display
  "EngSpd " : InportShadow
  Kp : Gain  Gain=0.04
  Logical Operator : Logic  Operator=OR  AllPortsSameDT=off  OutDataTypeStr=boolean
  Logical Operator1 : Logic  AllPortsSameDT=off  OutDataTypeStr=boolean
  Product : Product
  RPM Derating : Lookup_n-D  NumberOfTableDimensions=1  BreakpointsForDimension1=[0 1000 2000 3000 4000 5000 6000 7000]  Table=[1 1 1 1 1 1 1 0]  ExtrapMethod=Clip  UseLastTableValue=on  InternalRulePriority=Speed  RndMeth=Simplest  InputSameDT=on
  Relational Operator : RelationalOperator  Operator===  OutDataTypeStr=boolean  RndMeth=Nearest
  Relational Operator1 : RelationalOperator  Operator===  OutDataTypeStr=boolean  RndMeth=Nearest
  Saturation : Saturate  UpperLimit=100  LowerLimit=0
  Sum : Sum  Inputs=|+-
  Switch : Switch  Threshold=1
  TP : Outport
  wires:
  Switch/1 -> TP/1
  EngSpd/1 -> RPM Derating/1
  RPM Derating/1 -> Product/2  "2"
  Shifter/1 -> Relational Operator/2, Relational Operator1/1
  Constant/1 -> Relational Operator/1
  Constant1/1 -> Relational Operator1/2
  Relational Operator/1 -> Logical Operator/1
  Relational Operator1/1 -> Logical Operator/2
  Logical Operator/1 -> Logical Operator1/1
  Constant2/1 -> Sum/1
  "EngSpd "/1 -> Sum/2
  Sum/1 -> Kp/1
  Kp/1 -> Saturation/1
  Saturation/1 -> Switch/1
  Logical Operator1/1 -> Switch/2  "Idle"
  Compare To Constant1/1 -> Logical Operator1/2
  APP/1 -> Display/1, Based on APP to TP test data from 2013 Malibu1/1, Compare To Constant1/1  "3"
  Product/1 -> Switch/3
  Based on APP to TP test data from 2013 Malibu1/1 -> Product/1  "1"

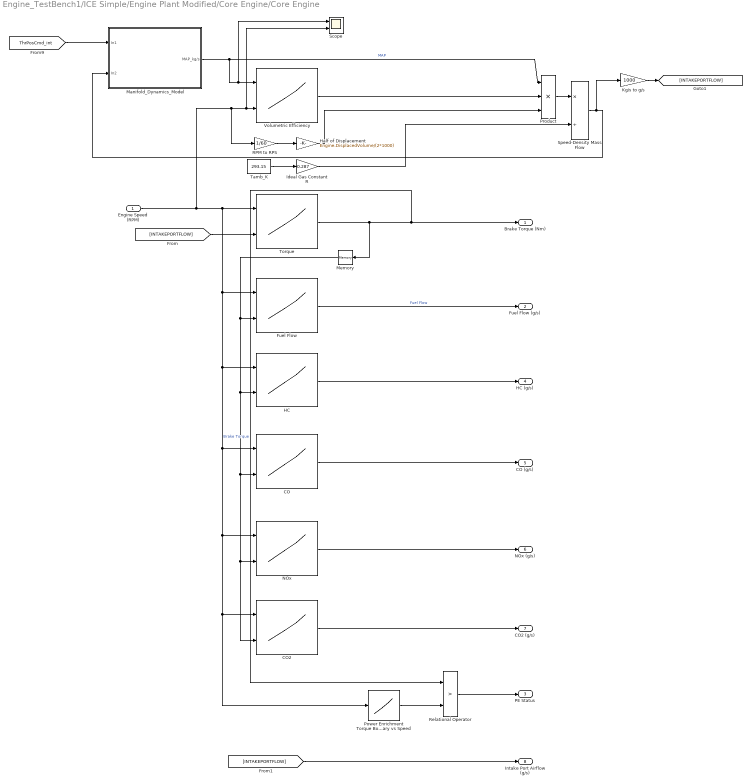
== system Engine_TestBench1/ICE Simple/Engine Plant Modified/Core Engine/Core Engine ==
  Engine Speed (RPM) : Inport
  CO : Lookup2D  RowIndex=Engine.Engine.Emissions.SPEED  ColumnIndex=Engine.Engine.Emissions.TQ  Table=Engine.Engine.Emissions.CO/1000  LookUpMeth=Interpolation-Use End Values
  CO2 : Lookup2D  RowIndex=Engine.Engine.Emissions.SPEED  ColumnIndex=Engine.Engine.Emissions.TQ  Table=Engine.Engine.Emissions.CO2/1000  LookUpMeth=Interpolation-Use End Values
  Fuel Flow : Lookup2D  RowIndex=Engine.Engine.FuelFlow.SPEED  ColumnIndex=Engine.Engine.FuelFlow.TQ  Table=Engine.Engine.FuelFlow.FuelFlow  LookUpMeth=Interpolation-Use End Values
  HC : Lookup2D  RowIndex=Engine.Engine.Emissions.SPEED  ColumnIndex=Engine.Engine.Emissions.TQ  Table=Engine.Engine.Emissions.HC/1000  LookUpMeth=Interpolation-Use End Values
  Half of Displacement : Gain  Gain=Engine.DisplacedVolume/(2*1000)
  Ideal Gas Constant R : Gain  Gain=0.287
  Kg/s to g/s : Gain  Gain=1000
  Manifold_Dynamics_Model : Subsystem
  Memory : Memory
  NOx : Lookup2D  RowIndex=Engine.Engine.Emissions.SPEED  ColumnIndex=Engine.Engine.Emissions.TQ  Table=Engine.Engine.Emissions.NOx/1000  LookUpMeth=Interpolation-Use End Values
  Power Enrichment Torque Boundary vs Speed : Lookup_n-D  NumberOfTableDimensions=1  BreakpointsForDimension1=Engine.Engine.PEBound.SPEED  Table=Engine.Engine.PEBound.PEBound  ExtrapMethod=Clip  InternalRulePriority=Speed  RndMeth=Simplest  InputSameDT=on
  Product : Product  Inputs=***
  RPM to RPS : Gain  Gain=1/60
  Relational Operator : RelationalOperator  Operator=>  OutDataTypeStr=boolean  ZeroCross=off  RndMeth=Nearest
  Scope : Scope  NumInputPorts=2
  Speed-Density Mass Flow : Product  Inputs=*/
  Tamb_K : Constant  Value=293.15
  Torque : Lookup2D  RowIndex=Engine.Engine.TQ.SPEED  ColumnIndex=Engine.Engine.TQ.MAF  Table=Engine.Engine.TQ.TQ  LookUpMeth=Interpolation-Use End Values
  Volumetric Efficiency : Lookup2D  RowIndex=Engine.Engine.VE.MAP  ColumnIndex=Engine.Engine.VE.SPEED  Table=Engine.Engine.VE.VE  LookUpMeth=Interpolation-Use End Values
  Brake Torque (Nm) : Outport
  Fuel Flow (g/s) : Outport  Port=2
  PE Status : Outport  Port=3
  HC (g/s) : Outport  Port=4
  CO (g/s) : Outport  Port=5
  NOx (g/s) : Outport  Port=6
  CO2 (g/s) : Outport  Port=7
  Intake Port Airflow (g/s) : Outport  Port=8
  wires:
  Torque/1 -> Brake Torque (Nm)/1, Relational Operator/1, Memory/1  "Brake Torque"
  [INTAKEPORTFLOW] -> Torque/2
  Fuel Flow/1 -> Fuel Flow (g/s)/1  "Fuel Flow"
  Memory/1 -> CO2/2, NOx/2, CO/2, HC/2, Fuel Flow/2
  Power Enrichment Torque Boundary vs Speed/1 -> Relational Operator/2
  Relational Operator/1 -> PE Status/1
  HC/1 -> HC (g/s)/1
  CO/1 -> CO (g/s)/1
  NOx/1 -> NOx (g/s)/1
  CO2/1 -> CO2 (g/s)/1
  [INTAKEPORTFLOW] -> Intake Port Airflow (g/s)/1
  Volumetric Efficiency/1 -> Product/2
  Ideal Gas Constant R/1 -> Speed-Density Mass Flow/2
  Product/1 -> Speed-Density Mass Flow/1
  Tamb_K/1 -> Ideal Gas Constant R/1
  RPM to RPS/1 -> Half of Displacement/1
  Half of Displacement/1 -> Product/3
  Engine Speed (RPM)/1 -> Torque/1, Fuel Flow/1, HC/1, CO/1, NOx/1, Power Enrichment Torque Boundary vs Speed/1, CO2/1, RPM to RPS/1, Scope/2, Volumetric Efficiency/2
  [ThrPosCmd_int] -> Manifold_Dynamics_Model/1(In1)
  Manifold_Dynamics_Model/1(MAP_kg/s) -> Product/1, Scope/1, Volumetric Efficiency/1  "MAP"
  Kg/s to g/s/1 -> [INTAKEPORTFLOW]
  Speed-Density Mass Flow/1 -> Manifold_Dynamics_Model/2(In2), Kg/s to g/s/1
